simulink model "gm_DVBS"  (R2023b)
settings: Solver=FixedStepAuto  StartTime=0.0  StopTime=160000/fs  FixedStep=5e-9  RelTol=1e-3  EnableMultiTasking=on
undefined symbols (not defined in the file or in its folder): ctrlIn, fc, fs, iniStates, k, n, oneData, rb, Rcos, simDataIn, sourceData
libraries: simulink x29, hdlsllib x23, commdigbbndpm3 x4, commhdlblkcod x4, dspsrcs4 x3, whdledac x1, commsink2 x1, commcnvintrlv2 x1, commchan3 x1, dsphdlsigops2 x1, commcnvcod2 x1
(part 2 of 2)

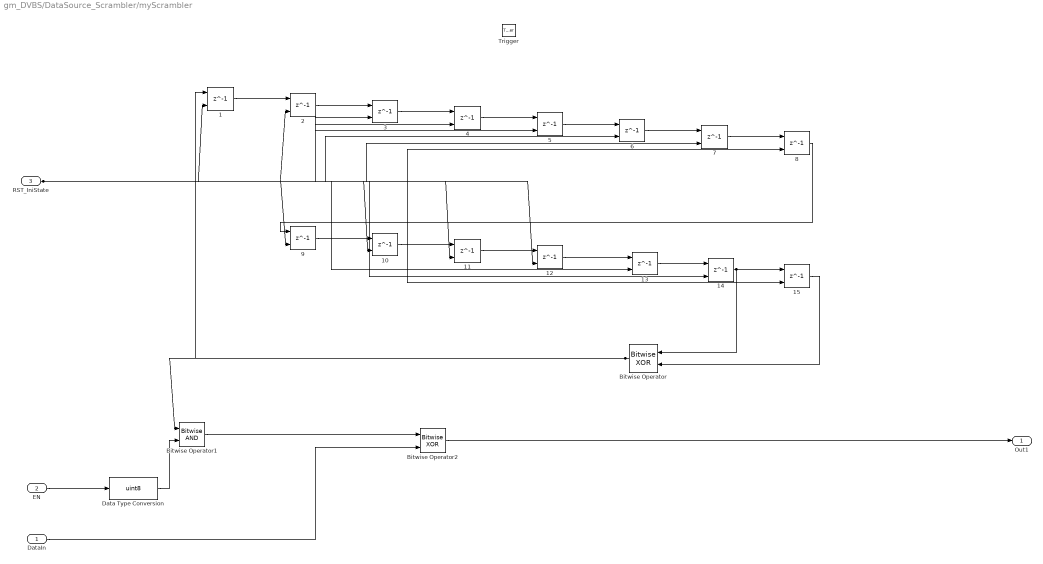
== system gm_DVBS/DataSource_Scrambler/myScrambler ==
  DataIn : Inport  OutDataTypeStr=uint8  PortDimensions=1
  EN : Inport  Port=2  OutDataTypeStr=boolean  PortDimensions=1
  RST_IniState : Inport  Port=3  OutDataTypeStr=boolean  PortDimensions=1
  Trigger : TriggerPort  VariantControl=(inherit)  PortDimensions=1  OutDataTypeStr=boolean
  1 : Delay  DelayLength=1  InitialCondition=iniStates(1)  ExternalReset=Level
      settings: InputPortMap=u0,r5
  10 : Delay  DelayLength=1  InitialCondition=iniStates(10)  ExternalReset=Level
      settings: InputPortMap=u0,r5
  11 : Delay  DelayLength=1  InitialCondition=iniStates(11)  ExternalReset=Level
      settings: InputPortMap=u0,r5
  12 : Delay  DelayLength=1  InitialCondition=iniStates(12)  ExternalReset=Level
      settings: InputPortMap=u0,r5
  13 : Delay  DelayLength=1  InitialCondition=iniStates(13)  ExternalReset=Level
      settings: InputPortMap=u0,r5
  14 : Delay  DelayLength=1  InitialCondition=iniStates(14)  ExternalReset=Level
      settings: InputPortMap=u0,r5
  15 : Delay  DelayLength=1  InitialCondition=iniStates(15)  ExternalReset=Level
      settings: InputPortMap=u0,r5
  2 : Delay  DelayLength=1  InitialCondition=iniStates(2)  ExternalReset=Level
      settings: InputPortMap=u0,r5
  3 : Delay  DelayLength=1  InitialCondition=iniStates(3)  ExternalReset=Level
      settings: InputPortMap=u0,r5
  4 : Delay  DelayLength=1  InitialCondition=iniStates(4)  ExternalReset=Level
      settings: InputPortMap=u0,r5
  5 : Delay  DelayLength=1  InitialCondition=iniStates(5)  ExternalReset=Level
      settings: InputPortMap=u0,r5
  6 : Delay  DelayLength=1  InitialCondition=iniStates(6)  ExternalReset=Level
      settings: InputPortMap=u0,r5
  7 : Delay  DelayLength=1  InitialCondition=iniStates(7)  ExternalReset=Level
      settings: InputPortMap=u0,r5
  8 : Delay  DelayLength=1  InitialCondition=iniStates(8)  ExternalReset=Level
      settings: InputPortMap=u0,r5
  9 : Delay  DelayLength=1  InitialCondition=iniStates(9)  ExternalReset=Level
      settings: InputPortMap=u0,r5
  Bitwise Operator : simulink/Logic and Bit Operations/Bitwise Operator  logicop=XOR  UseBitMask=off  NumInputPorts=2  BitMask=bin2dec('11011001')  BitMaskRealWorld=Stored Integer
  Bitwise Operator1 : simulink/Logic and Bit Operations/Bitwise Operator  logicop=AND  UseBitMask=off  NumInputPorts=2  BitMask=bin2dec('11011001')  BitMaskRealWorld=Stored Integer
  Bitwise Operator2 : simulink/Logic and Bit Operations/Bitwise Operator  logicop=XOR  UseBitMask=off  NumInputPorts=2  BitMask=bin2dec('11011001')  BitMaskRealWorld=Stored Integer
  Data Type Conversion : DataTypeConversion  OutDataTypeStr=uint8  SaturateOnIntegerOverflow=off  RndMeth=Floor
  Out1 : Outport  InitialOutput=0
  wires:
  DataIn/1 -> Bitwise Operator2/2
  EN/1 -> Data Type Conversion/1
  RST_IniState/1 -> 14/2, 13/2, 12/2, 11/2, 10/2, 9/2, 8/2, 7/2, 6/2, 5/2, 4/2, 3/2, 2/2, 1/2, 15/2
  Bitwise Operator/1 -> Bitwise Operator1/1, 1/1
  Bitwise Operator1/1 -> Bitwise Operator2/1
  Bitwise Operator2/1 -> Out1/1
  Data Type Conversion/1 -> Bitwise Operator1/2
  15/1 -> Bitwise Operator/2
  1/1 -> 2/1
  2/1 -> 3/1
  3/1 -> 4/1
  4/1 -> 5/1
  5/1 -> 6/1
  6/1 -> 7/1
  7/1 -> 8/1
  8/1 -> 9/1
  9/1 -> 10/1
  10/1 -> 11/1
  11/1 -> 12/1
  12/1 -> 13/1
  13/1 -> 14/1
  14/1 -> Bitwise Operator/1, 15/1

== system gm_DVBS/DataSource_Scrambler/sigSource ==
  DataGenEn : Inport  OutDataTypeStr=boolean  PortDimensions=1  SampleTime=5e-09
  Enable : Inport  Port=2  OutDataTypeStr=boolean  SampleTime=5e-09
  1-D Lookup Table : Lookup_n-D  NumberOfTableDimensions=1  LookupTableObject=''  BreakpointsForDimension1=[0:18800-1]'  BreakpointsForDimension1FirstPoint=10  BreakpointsForDimension2FirstPoint=10  BreakpointsForDimension1Spacing=12  BreakpointsForDimension2Spacing=12  IndexSearchMethod=Evenly spaced points  Table=sourceData  InterpMethod=Flat  DiagnosticForOutOfRangeInput=Error  InternalRulePriority=Speed  OutDataTypeStr=uint8  RndMeth=Simplest
  DATA_IN : DataTypeConversion  OutDataTypeStr=fixdt(0,8,0)
  HDL Counter : Subsystem
      settings: MinAlgLoopOccurrences=on
  RS_Gen : Subsystem
  out_0_pipe : Delay  DelayLength=double(1)  InitialCondition=0
  out_1_pipe : Delay  DelayLength=double(1)  InitialCondition=0
  out_2_pipe : Delay  DelayLength=double(1)  InitialCondition=0
  out_3_pipe : Delay  DelayLength=double(1)  InitialCondition=0
  simStart : Outport  SampleTime=5e-09  InitialOutput=0
  simEnd : Outport  Port=2  SampleTime=5e-09  InitialOutput=0
  simEN : Outport  Port=3  SampleTime=5e-09  InitialOutput=0
  simDataIn : Outport  Port=4  SampleTime=5e-09  InitialOutput=0
  wires:
  Enable/1 -> HDL Counter/Enable, RS_Gen/1(Enable_out2)
  DataGenEn/1 -> HDL Counter/1(in0)
  1-D Lookup Table/1 -> DATA_IN/1
  DATA_IN/1 -> out_3_pipe/1
  HDL Counter/1(out0) -> 1-D Lookup Table/1
  RS_Gen/1(simStart) -> out_0_pipe/1
  RS_Gen/2(simEnd) -> out_1_pipe/1
  RS_Gen/3(simEN) -> out_2_pipe/1
  out_0_pipe/1 -> simStart/1
  out_1_pipe/1 -> simEnd/1
  out_2_pipe/1 -> simEN/1
  out_3_pipe/1 -> simDataIn/1

== system gm_DVBS/DataSource_Scrambler1/CLKdivide ==
  Constant : Constant  Value=8  VectorParams1D=off  OutDataTypeStr=uint8  SampleTime=1/fs
  Constant1 : Constant  Value=25  VectorParams1D=off  OutDataTypeStr=uint8  SampleTime=1/fs
  Delay : Delay  DelayLength=1
  Detect Rise Positive : hdlsllib/Logic and Bit Operations/Detect Rise Positive  vinit=0  OutDataTypeStr=boolean
  HDL Counter : hdlsllib/Sources/HDL Counter  CountType=Count limited  CountInit=1  CountStep=1  CountMax=8  CountFromType=Initial value  CountFrom=1  CountResetPort=off  CountLoadPort=off  CountEnbPort=on  CountDirPort=off  CountHitOutputPort=off  CountDataType=Unsigned  CountWordLen=8  CountFracLen=0  CountSampTime=1
  HDL Counter2 : hdlsllib/Sources/HDL Counter  CountType=Count limited  CountInit=1  CountStep=1  CountMax=25  CountFromType=Initial value  CountFrom=1  CountResetPort=off  CountLoadPort=off  CountEnbPort=off  CountDirPort=off  CountHitOutputPort=off  CountDataType=Unsigned  CountWordLen=8  CountFracLen=0  CountSampTime=1/fs
  Relational Operator : RelationalOperator  Operator===  OutDataTypeStr=boolean  InputSameDT=off
  Relational Operator1 : RelationalOperator  Operator===  OutDataTypeStr=boolean  InputSameDT=off
  DataGenEn : Outport  VectorParamsAs1DForOutWhenUnconnected=off
  BinEn : Outport  Port=2  VectorParamsAs1DForOutWhenUnconnected=off
  wires:
  Constant/1 -> Relational Operator1/2
  Detect Rise Positive/1 -> DataGenEn/1
  Relational Operator1/1 -> Detect Rise Positive/1
  HDL Counter/1 -> Relational Operator1/1
  HDL Counter2/1 -> Relational Operator/1
  Delay/1 -> BinEn/1
  Relational Operator/1 -> HDL Counter/1, Delay/1
  Constant1/1 -> Relational Operator/2

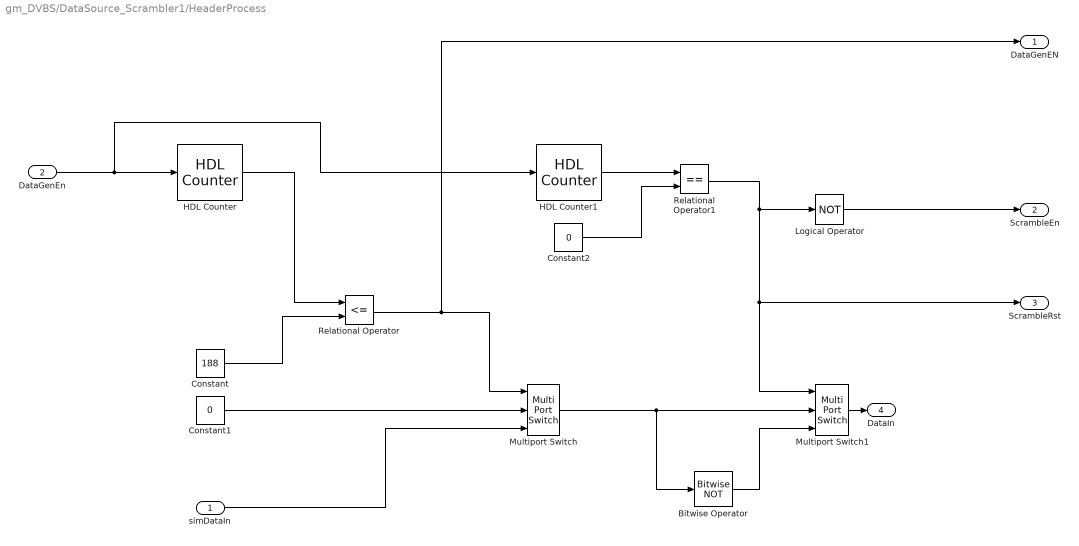
== system gm_DVBS/DataSource_Scrambler1/HeaderProcess ==
  simDataIn : Inport
  DataGenEn : Inport  Port=2
  Bitwise Operator : simulink/Logic and Bit Operations/Bitwise Operator  logicop=NOT  UseBitMask=off  BitMask=bin2dec('11011001')  BitMaskRealWorld=Stored Integer
  Constant : Constant  Value=188  OutDataTypeStr=uint8  SampleTime=1/fs
  Constant1 : Constant  Value=0  OutDataTypeStr=uint8
  Constant2 : Constant  Value=0  OutDataTypeStr=uint8
  HDL Counter : hdlsllib/Sources/HDL Counter  CountType=Count limited  CountInit=1  CountStep=1  CountMax=n  CountFromType=Initial value  CountFrom=1  CountResetPort=off  CountLoadPort=off  CountEnbPort=on  CountDirPort=off  CountHitOutputPort=off  CountDataType=Unsigned  CountWordLen=8  CountFracLen=0  CountSampTime=1/fs
  HDL Counter1 : hdlsllib/Sources/HDL Counter  CountType=Count limited  CountInit=0  CountStep=1  CountMax=n*8-1  CountFromType=Initial value  CountFrom=0  CountResetPort=off  CountLoadPort=off  CountEnbPort=on  CountDirPort=off  CountHitOutputPort=off  CountDataType=Unsigned  CountWordLen=16  CountFracLen=0  CountSampTime=1/fs
  Logical Operator : Logic  Operator=NOT  AllPortsSameDT=off  OutDataTypeStr=boolean
  Multiport Switch : MultiPortSwitch  DataPortOrder=Specify indices  DataPortIndices={0,1}  OutDataTypeStr=uint8  SaturateOnIntegerOverflow=off  InputSameDT=off
  Multiport Switch1 : MultiPortSwitch  DataPortOrder=Specify indices  DataPortIndices={0,1}  OutDataTypeStr=uint8  SaturateOnIntegerOverflow=off  InputSameDT=off
  Relational Operator : RelationalOperator  Operator=<=  OutDataTypeStr=boolean  InputSameDT=off
  Relational Operator1 : RelationalOperator  Operator===  OutDataTypeStr=boolean  InputSameDT=off
  DataGenEN : Outport  VectorParamsAs1DForOutWhenUnconnected=off
  ScrambleEn : Outport  Port=2  VectorParamsAs1DForOutWhenUnconnected=off
  ScrambleRst : Outport  Port=3  VectorParamsAs1DForOutWhenUnconnected=off
  DataIn : Outport  Port=4
  wires:
  DataGenEn/1 -> HDL Counter/1, HDL Counter1/1
  simDataIn/1 -> Multiport Switch/3
  Logical Operator/1 -> ScrambleEn/1
  Constant1/1 -> Multiport Switch/2
  Constant2/1 -> Relational Operator1/2
  Constant/1 -> Relational Operator/2
  Relational Operator1/1 -> Logical Operator/1, Multiport Switch1/1, ScrambleRst/1
  Relational Operator/1 -> Multiport Switch/1, DataGenEN/1
  HDL Counter1/1 -> Relational Operator1/1
  HDL Counter/1 -> Relational Operator/1
  Multiport Switch/1 -> Multiport Switch1/2, Bitwise Operator/1
  Bitwise Operator/1 -> Multiport Switch1/3
  Multiport Switch1/1 -> DataIn/1

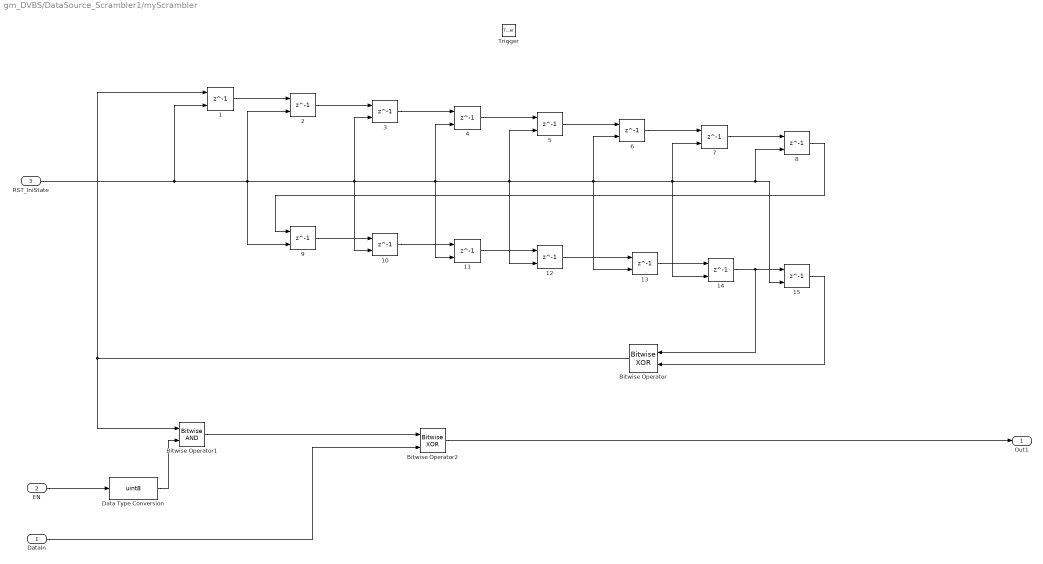
== system gm_DVBS/DataSource_Scrambler1/myScrambler ==
  DataIn : Inport  OutDataTypeStr=uint8
  EN : Inport  Port=2  OutDataTypeStr=boolean
  RST_IniState : Inport  Port=3  OutDataTypeStr=boolean
  Trigger : TriggerPort  VariantControl=Variant  PortDimensions=1
  1 : Delay  DelayLength=1  InitialCondition=iniStates(1)  ExternalReset=Level
      settings: InputPortMap=u0,r5
  10 : Delay  DelayLength=1  InitialCondition=iniStates(10)  ExternalReset=Level
      settings: InputPortMap=u0,r5
  11 : Delay  DelayLength=1  InitialCondition=iniStates(11)  ExternalReset=Level
      settings: InputPortMap=u0,r5
  12 : Delay  DelayLength=1  InitialCondition=iniStates(12)  ExternalReset=Level
      settings: InputPortMap=u0,r5
  13 : Delay  DelayLength=1  InitialCondition=iniStates(13)  ExternalReset=Level
      settings: InputPortMap=u0,r5
  14 : Delay  DelayLength=1  InitialCondition=iniStates(14)  ExternalReset=Level
      settings: InputPortMap=u0,r5
  15 : Delay  DelayLength=1  InitialCondition=iniStates(15)  ExternalReset=Level
      settings: InputPortMap=u0,r5
  2 : Delay  DelayLength=1  InitialCondition=iniStates(2)  ExternalReset=Level
      settings: InputPortMap=u0,r5
  3 : Delay  DelayLength=1  InitialCondition=iniStates(3)  ExternalReset=Level
      settings: InputPortMap=u0,r5
  4 : Delay  DelayLength=1  InitialCondition=iniStates(4)  ExternalReset=Level
      settings: InputPortMap=u0,r5
  5 : Delay  DelayLength=1  InitialCondition=iniStates(5)  ExternalReset=Level
      settings: InputPortMap=u0,r5
  6 : Delay  DelayLength=1  InitialCondition=iniStates(6)  ExternalReset=Level
      settings: InputPortMap=u0,r5
  7 : Delay  DelayLength=1  InitialCondition=iniStates(7)  ExternalReset=Level
      settings: InputPortMap=u0,r5
  8 : Delay  DelayLength=1  InitialCondition=iniStates(8)  ExternalReset=Level
      settings: InputPortMap=u0,r5
  9 : Delay  DelayLength=1  InitialCondition=iniStates(9)  ExternalReset=Level
      settings: InputPortMap=u0,r5
  Bitwise Operator : simulink/Logic and Bit Operations/Bitwise Operator  logicop=XOR  UseBitMask=off  NumInputPorts=2  BitMask=bin2dec('11011001')  BitMaskRealWorld=Stored Integer
  Bitwise Operator1 : simulink/Logic and Bit Operations/Bitwise Operator  logicop=AND  UseBitMask=off  NumInputPorts=2  BitMask=bin2dec('11011001')  BitMaskRealWorld=Stored Integer
  Bitwise Operator2 : simulink/Logic and Bit Operations/Bitwise Operator  logicop=XOR  UseBitMask=off  NumInputPorts=2  BitMask=bin2dec('11011001')  BitMaskRealWorld=Stored Integer
  Data Type Conversion : DataTypeConversion  OutDataTypeStr=uint8  SaturateOnIntegerOverflow=off  RndMeth=Floor
  Out1 : Outport  InitialOutput=0
  wires:
  Data Type Conversion/1 -> Bitwise Operator1/2
  RST_IniState/1 -> 3/2, 5/2, 6/2, 7/2, 15/2, 8/2, 14/2, 13/2, 12/2, 11/2, 4/2, 10/2, 9/2, 2/2, 1/2
  8/1 -> 9/1
  Bitwise Operator2/1 -> Out1/1
  DataIn/1 -> Bitwise Operator2/2
  Bitwise Operator1/1 -> Bitwise Operator2/1
  EN/1 -> Data Type Conversion/1
  Bitwise Operator/1 -> 1/1, Bitwise Operator1/1
  15/1 -> Bitwise Operator/2
  14/1 -> 15/1, Bitwise Operator/1
  13/1 -> 14/1
  12/1 -> 13/1
  11/1 -> 12/1
  10/1 -> 11/1
  9/1 -> 10/1
  7/1 -> 8/1
  6/1 -> 7/1
  5/1 -> 6/1
  4/1 -> 5/1
  3/1 -> 4/1
  2/1 -> 3/1
  1/1 -> 2/1

== system gm_DVBS/DataSource_Scrambler1/sigSource ==
  DataGenEn : Inport
  Enable : EnablePort
  1-D Lookup Table : Lookup_n-D  NumberOfTableDimensions=1  LookupTableObject=''  BreakpointsForDimension1=[0:18800-1]'  BreakpointsForDimension1FirstPoint=10  BreakpointsForDimension2FirstPoint=10  BreakpointsForDimension1Spacing=12  BreakpointsForDimension2Spacing=12  IndexSearchMethod=Evenly spaced points  Table=sourceData  InterpMethod=Flat  DiagnosticForOutOfRangeInput=Error  InternalRulePriority=Speed  OutDataTypeStr=uint8  RndMeth=Simplest
  DATA_IN : DataTypeConversion  OutDataTypeStr=inDataType  SaturateOnIntegerOverflow=off  RndMeth=Floor
  Detect Rise Positive : hdlsllib/Logic and Bit Operations/Detect Rise Positive  vinit=0  OutDataTypeStr=boolean
  Detect Rise Positive1 : hdlsllib/Logic and Bit Operations/Detect Rise Positive  vinit=0  OutDataTypeStr=boolean
  HDL Counter : hdlsllib/Sources/HDL Counter  CountType=Count limited  CountInit=0  CountStep=1  CountMax=18800-1  CountFromType=Initial value  CountFrom=0  CountResetPort=off  CountLoadPort=off  CountEnbPort=on  CountDirPort=off  CountHitOutputPort=off  CountDataType=Unsigned  CountWordLen=32  CountFracLen=0  CountSampTime=1/fs
  RS_Gen : Subsystem
  Subsystem : Subsystem  Commented=on
  simStart : Outport  InitialOutput=0
  simEnd : Outport  Port=2  InitialOutput=0
  simEN : Outport  Port=3  InitialOutput=0
  simDataIn : Outport  Port=4  InitialOutput=0
  wires:
  Detect Rise Positive1/1 -> simEnd/1
  Detect Rise Positive/1 -> simStart/1
  DATA_IN/1 -> simDataIn/1
  RS_Gen/3(simEN) -> simEN/1
  RS_Gen/2(simEnd) -> Detect Rise Positive1/1
  RS_Gen/1(simStart) -> Detect Rise Positive/1
  DataGenEn/1 -> RS_Gen/Trigger, HDL Counter/1
  HDL Counter/1 -> 1-D Lookup Table/1
  1-D Lookup Table/1 -> DATA_IN/1

== system gm_DVBS/Interleaver/Con_Interleaver ==
  In1 : Inport
  Trigger : TriggerPort  VariantControl=Variant  PortDimensions=1
  Convolutional Interleaver : commcnvintrlv2/Convolutional Interleaver  N=12  B=17  ic=0
      settings: LibrarySourceBlock=|
      | commhdlinterleave/Convolutional
      | Interleaver
  Out1 : Outport  InitialOutput=0
  wires:
  Convolutional Interleaver/1 -> Out1/1
  In1/1 -> Convolutional Interleaver/1

== system gm_DVBS/QPSK/QPSK_Modulation ==
  In1 : Inport
  Add : Sum  Inputs=+-
  Complex to Real-Imag : ComplexToRealImag
  Cosine : Sin  Frequency=fc*2*pi  Phase=pi/2  SampleTime=1/fs
  Discrete FIR Filter : DiscreteFir  Coefficients=Rcos
  Discrete FIR Filter1 : DiscreteFir  Coefficients=Rcos
  Product : Product
  Product1 : Product
  QPSK Modulator Baseband : commdigbbndpm3/QPSK Modulator Baseband  InType=Bit  Enc=Gray  Ph=pi/4  outDtype=double  outWordLen=16  outUDDataType=sfix(16)  outFracLenMode=Best precision  outFracLen=15  outDataTypeStr=double  outLastDataTypeStr=double
      settings: LibrarySourceBlock=|
      | commhdldigbbndpm/QPSK
      | Modulator
      | Baseband
  Sign : Signum  Commented=through
  Sign1 : Signum  Commented=through
  Sine : Sin  Frequency=fc*2*pi  SampleTime=1/fs
  Out1 : Outport
  Out2 : Outport  Port=2  VectorParamsAs1DForOutWhenUnconnected=off
  wires:
  In1/1 -> QPSK Modulator Baseband/1
  Sign1/1 -> Discrete FIR Filter1/1
  Complex to Real-Imag/1 -> Sign/1
  Discrete FIR Filter/1 -> Product/1
  Add/1 -> Out1/1
  QPSK Modulator Baseband/1 -> Complex to Real-Imag/1, Out2/1
  Product/1 -> Add/1
  Product1/1 -> Add/2
  Discrete FIR Filter1/1 -> Product1/2
  Sign/1 -> Discrete FIR Filter/1
  Sine/1 -> Product1/1
  Cosine/1 -> Product/2
  Complex to Real-Imag/2 -> Sign1/1

== system gm_DVBS/QPSK/Subsystem ==
  In1 : Inport
  Cos : Sin  Frequency=fc*2*pi  Phase=pi/2  SampleTime=1/fs
  Discrete FIR Filter : DiscreteFir  Coefficients=Rcos
  Discrete FIR Filter1 : DiscreteFir  Coefficients=Rcos
  Product : Product
  Product1 : Product
  QPSK Demodulator Baseband : commdigbbndpm3/QPSK Demodulator Baseband  OutType=Integer  DecType=Hard decision  VarSource=Dialog  Variance=1  Dec=Gray  Ph=pi/4  outDtype1=Inherit via internal rule  outDtype2=Inherit via internal rule  derotateFactorWordLen=16  derotateFactorDataTypeStr=Inherit: Same word length as input  derotateFactorLastDataTypeStr=Inherit: Same word length as input
      settings: LibrarySourceBlock=|
      | commhdldigbbndpm/QPSK
      | Demodulator
      | Baseband
  Real-Imag to Complex : RealImagToComplex
  Sin : Sin  Frequency=fc*2*pi  SampleTime=1/fs
  Out1 : Outport
  wires:
  Discrete FIR Filter/1 -> Real-Imag to Complex/2
  Discrete FIR Filter1/1 -> Real-Imag to Complex/1
  QPSK Demodulator Baseband/1 -> Out1/1
  Real-Imag to Complex/1 -> QPSK Demodulator Baseband/1
  Product1/1 -> Discrete FIR Filter/1
  Product/1 -> Discrete FIR Filter1/1
  Sin/1 -> Product1/1
  Cos/1 -> Product/2
  In1/1 -> Product/1, Product1/2

== system gm_DVBS/RS_Enc/RS ==
  RS_In : Inport  OutDataTypeStr=uint8
  RS_Start : Inport  Port=2  OutDataTypeStr=boolean
  RS_End : Inport  Port=3  OutDataTypeStr=boolean
  RS_VLD : Inport  Port=4  OutDataTypeStr=boolean
  Trigger : TriggerPort  VariantControl=Variant  PortDimensions=1
  Integer-Input RS Encoder HDL Optimized : commhdlblkcod/Integer-Input RS Encoder HDL Optimized  CodewordLength=n  MessageLength=k  PrimitivePolynomialSource=Property  PrimitivePolynomial=[1 0 0 0 1 1 1 0 1]  PuncturePatternSource=None  PuncturePattern=[ ones( 2, 1 ); zeros( 2, 1 ) ]  BSource=Property  B=0  SimulateUsing=Code generation
  Terminator : Terminator
  Terminator1 : Terminator
  Terminator2 : Terminator
  RS_Out : Outport  OutDataTypeStr=uint8  InitialOutput=0
  wires:
  Integer-Input RS Encoder HDL Optimized/4 -> Terminator2/1
  Integer-Input RS Encoder HDL Optimized/3 -> Terminator1/1
  Integer-Input RS Encoder HDL Optimized/2 -> Terminator/1
  RS_VLD/1 -> Integer-Input RS Encoder HDL Optimized/4
  RS_End/1 -> Integer-Input RS Encoder HDL Optimized/3
  RS_Start/1 -> Integer-Input RS Encoder HDL Optimized/2
  Integer-Input RS Encoder HDL Optimized/1 -> RS_Out/1
  RS_In/1 -> Integer-Input RS Encoder HDL Optimized/1

== system gm_DVBS/Subsystem/Subsystem ==
  Constant : Constant  OutDataTypeStr=boolean  SampleTime=1/fs
  NCO : dsphdlsigops2/NCO  PhaseIncrementSource=Property  PhaseIncrement=phInc  PhaseOffsetSource=Property  PhaseOffset=0  DitherSource=Property  NumDitherBits=4  SamplesPerFrame=1  LUTCompress=on  ResetAction=off  Waveform=Sine and cosine  PhasePort=off  SimulateUsing=Code generation  AccumulatorWL=N  PhaseQuantization=on  NumQuantizerAccumulatorBits=Q  OutputDataType=Binary point scaling  OutputWL=32  OutputFL=30
      settings: LibrarySourceBlock=dsphdlsrcs2/NCO
  sin : Outport
  cos : Outport  Port=2
  vld : Outport  Port=3
  wires:
  NCO/2 -> cos/1
  NCO/3 -> vld/1
  NCO/1 -> sin/1
  Constant/1 -> NCO/1

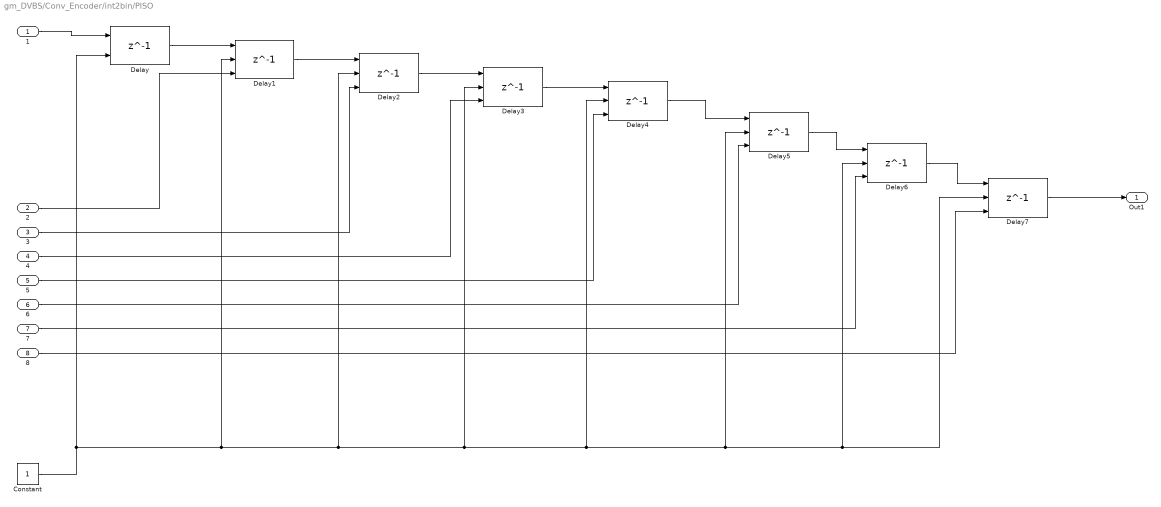
== system gm_DVBS/Conv_Encoder/int2bin/PISO ==
  1 : Inport
  2 : Inport  Port=2
  3 : Inport  Port=3
  4 : Inport  Port=4
  5 : Inport  Port=5
  6 : Inport  Port=6
  7 : Inport  Port=7
  8 : Inport  Port=8
  Constant : Constant  OutDataTypeStr=boolean  SampleTime=1
  Delay : Delay  DelayLength=1  InitialCondition=0  ShowEnablePort=on  UseCircularBuffer=on  SampleTime=1
      settings: InputPortMap=u0,e6
  Delay{1..7} (7 alike) : Delay  DelayLength=1  InitialConditionSource=Input port  InitialCondition=0  ShowEnablePort=on  UseCircularBuffer=on  SampleTime=1
      settings: InputPortMap=u0,e6,p4
  Out1 : Outport
  wires:
  5/1 -> Delay4/3
  Delay7/1 -> Out1/1
  Delay6/1 -> Delay7/1
  6/1 -> Delay5/3
  8/1 -> Delay7/3
  7/1 -> Delay6/3
  Delay4/1 -> Delay5/1
  Delay5/1 -> Delay6/1
  Constant/1 -> Delay3/2, Delay7/2, Delay6/2, Delay5/2, Delay4/2, Delay2/2, Delay1/2, Delay/2
  Delay3/1 -> Delay4/1
  4/1 -> Delay3/3
  3/1 -> Delay2/3
  2/1 -> Delay1/3
  Delay2/1 -> Delay3/1
  Delay1/1 -> Delay2/1
  Delay/1 -> Delay1/1
  1/1 -> Delay/1

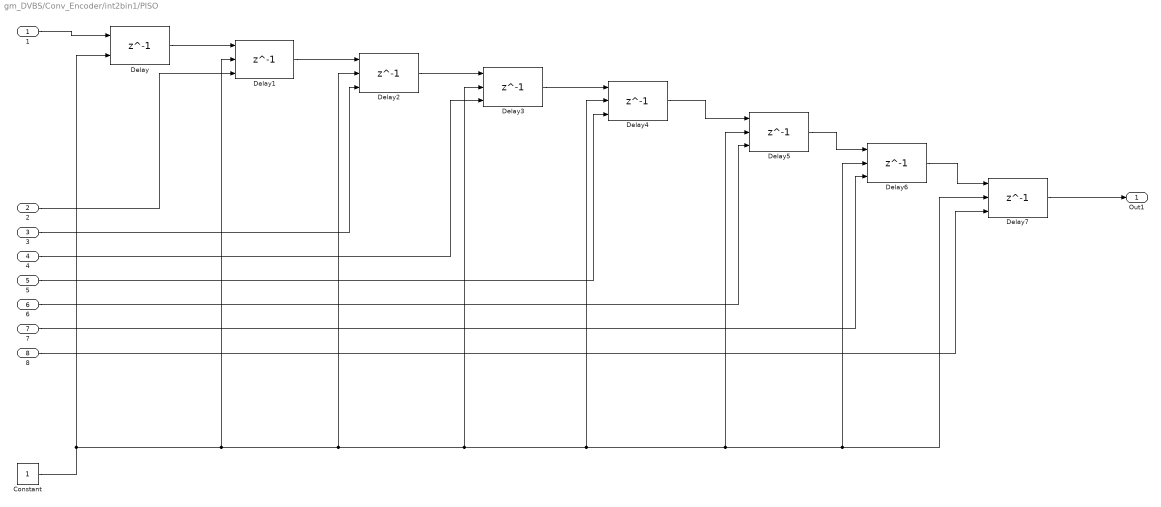
== system gm_DVBS/Conv_Encoder/int2bin1/PISO ==
  1 : Inport
  2 : Inport  Port=2
  3 : Inport  Port=3
  4 : Inport  Port=4
  5 : Inport  Port=5
  6 : Inport  Port=6
  7 : Inport  Port=7
  8 : Inport  Port=8
  Constant : Constant  OutDataTypeStr=boolean  SampleTime=1
  Delay : Delay  DelayLength=1  InitialCondition=0  ShowEnablePort=on  UseCircularBuffer=on  SampleTime=1
      settings: InputPortMap=u0,e6
  Delay{1..7} (7 alike) : Delay  DelayLength=1  InitialConditionSource=Input port  InitialCondition=0  ShowEnablePort=on  UseCircularBuffer=on  SampleTime=1
      settings: InputPortMap=u0,e6,p4
  Out1 : Outport
  wires:
  5/1 -> Delay4/3
  Delay7/1 -> Out1/1
  Delay6/1 -> Delay7/1
  6/1 -> Delay5/3
  8/1 -> Delay7/3
  7/1 -> Delay6/3
  Delay4/1 -> Delay5/1
  Delay5/1 -> Delay6/1
  Constant/1 -> Delay3/2, Delay7/2, Delay6/2, Delay5/2, Delay4/2, Delay2/2, Delay1/2, Delay/2
  Delay3/1 -> Delay4/1
  4/1 -> Delay3/3
  3/1 -> Delay2/3
  2/1 -> Delay1/3
  Delay2/1 -> Delay3/1
  Delay1/1 -> Delay2/1
  Delay/1 -> Delay1/1
  1/1 -> Delay/1

== system gm_DVBS/DataSource_Scrambler/CLKdivide/Detect Rise Positive ==
  note: Edge
  note: U(k)
  U : Inport  OutDataTypeStr=boolean  SampleTime=5e-09
  Delay Input1 : UnitDelay  Description=Store in Global RAM  DisableCoverage=on  InitialCondition=vinit  SampleTime=-1  HasFrameUpgradeWarning=on
  FixPt Relational Operator : RelationalOperator  Operator=>  OutDataTypeStr=boolean  ZeroCross=off  InputSameDT=off
  Positive : Subsystem  mask(Compare To Zero){relop=>, OutDataTypeStr=boolean, ZeroCross=off}
      mask prompts: relop "Simulink:masks:Operator_MP"; OutDataTypeStr "Simulink:masks:OutputDataType_MP"; ZeroCross "Simulink:masks:EnableZerocrossingDetection_MP"
      mask help: Simulink:masks:CompareToZero_MD
      mask init:
      | OutDataTypeStr = 'boolean';
      | ZeroCross = 'off';
      | blkName = 'DVBS/DataSource_Scrambler/CLKdivide/Detect Rise\nPositive/Positive';
      | relop = '>';
      | setValue = 'boolean';
      mask TypeOptions relop: == | ~= | < | <= | >= | >
      mask TypeOptions OutDataTypeStr: Simulink:masks:uint8 | Simulink:masks:boolean
      mask Callback ZeroCross: sl('zeroCrossEnable', gcbh);
      mask Display: disp([relop,' 0'])
  Y : Outport  SampleTime=5e-09
  wires:
  U/1 -> Positive/1(u)
  Delay Input1/1 -> FixPt Relational Operator/2
  FixPt Relational Operator/1 -> Y/1
  Positive/1(y) -> FixPt Relational Operator/1, Delay Input1/1

== system gm_DVBS/DataSource_Scrambler/Detect Rise Positive/Positive ==
  u : Inport  OutDataTypeStr=boolean  SampleTime=5e-09
  Compare : RelationalOperator  Operator=>  OutDataTypeStr=boolean  ZeroCross=off
  Constant : Constant  DisableCoverage=on  Value=0  OutDataTypeStr=Inherit: Inherit via back propagation  SampleTime=-1  PreserveConstantTs=on
  y : Outport  SampleTime=5e-09
  wires:
  u/1 -> Compare/1
  Compare/1 -> y/1
  Constant/1 -> Compare/2

== system gm_DVBS/DataSource_Scrambler/Detect Rise Positive1/Positive ==
  u : Inport  OutDataTypeStr=boolean  SampleTime=5e-09
  Compare : RelationalOperator  Operator=>  OutDataTypeStr=boolean  ZeroCross=off
  Constant : Constant  DisableCoverage=on  Value=0  OutDataTypeStr=Inherit: Inherit via back propagation  SampleTime=-1  PreserveConstantTs=on
  y : Outport  SampleTime=5e-09
  wires:
  u/1 -> Compare/1
  Compare/1 -> y/1
  Constant/1 -> Compare/2

== system gm_DVBS/DataSource_Scrambler/sigSource/HDL Counter ==
  in0 : Inport  OutDataTypeStr=boolean  SampleTime=5e-09
  Enable_out2 : EnablePort  OutDataTypeStr=boolean
  HDL Counter : hdlsllib/Sources/HDL Counter  CountType=Count limited  CountInit=0  CountStep=1  CountMax=18800-1  CountFromType=Initial value  CountFrom=0  CountResetPort=off  CountLoadPort=off  CountEnbPort=on  CountDirPort=off  CountHitOutputPort=off  CountDataType=Unsigned  CountWordLen=32  CountFracLen=0  CountSampTime=1/fs
  out0 : Outport  OutDataTypeStr=uint32  SampleTime=5e-09  InitialOutput=0
  wires:
  HDL Counter/1 -> out0/1
  in0/1 -> HDL Counter/1

== system gm_DVBS/DataSource_Scrambler/sigSource/RS_Gen ==
  Enable_out2 : Inport  OutDataTypeStr=boolean  SampleTime=5e-09
  Constant : Constant  Value=188  OutDataTypeStr=uint16  SampleTime=5e-09
  DATA_IN1 : DataTypeConversion  OutDataTypeStr=boolean  SampleTime=5e-09  SaturateOnIntegerOverflow=off  RndMeth=Floor
  DATA_IN2 : DataTypeConversion  OutDataTypeStr=boolean  SampleTime=5e-09  SaturateOnIntegerOverflow=off  RndMeth=Floor
  DATA_IN3 : DataTypeConversion  OutDataTypeStr=boolean  SampleTime=5e-09  SaturateOnIntegerOverflow=off  RndMeth=Floor
  MATLAB Function : Subsystem
      settings: MinAlgLoopOccurrences=on
  simStart : Outport  SampleTime=5e-09  InitialOutput=0
  simEnd : Outport  Port=2  SampleTime=5e-09  InitialOutput=0
  simEN : Outport  Port=3  SampleTime=5e-09  InitialOutput=0
  wires:
  Constant/1 -> MATLAB Function/1(in0)
  DATA_IN1/1 -> simEN/1
  DATA_IN2/1 -> simStart/1
  DATA_IN3/1 -> simEnd/1
  MATLAB Function/1(out0) -> DATA_IN1/1
  MATLAB Function/2(out1) -> DATA_IN2/1
  MATLAB Function/3(out2) -> DATA_IN3/1
  Enable_out2/1 -> MATLAB Function/Enable

== system gm_DVBS/DataSource_Scrambler1/sigSource/RS_Gen ==
  Trigger : TriggerPort  VariantControl=(inherit)  PortDimensions=1
  Constant : Constant  Value=204  OutDataTypeStr=uint16  SampleTime=-1
  DATA_IN1 : DataTypeConversion  OutDataTypeStr=boolean  SaturateOnIntegerOverflow=off  RndMeth=Floor
  DATA_IN2 : DataTypeConversion  OutDataTypeStr=boolean  SaturateOnIntegerOverflow=off  RndMeth=Floor
  DATA_IN3 : DataTypeConversion  OutDataTypeStr=boolean  SaturateOnIntegerOverflow=off  RndMeth=Floor
  MATLAB Function : MATLAB Function  TreatAsAtomicUnit=on
  simStart : Outport  InitialOutput=0
  simEnd : Outport  Port=2  InitialOutput=0
  simEN : Outport  Port=3  InitialOutput=0
  wires:
  MATLAB Function/1(enable) -> DATA_IN1/1
  Constant/1 -> MATLAB Function/1(totalLength)
  DATA_IN2/1 -> simStart/1
  DATA_IN1/1 -> simEN/1
  DATA_IN3/1 -> simEnd/1
  MATLAB Function/2(start) -> DATA_IN2/1
  MATLAB Function/3(endSignal) -> DATA_IN3/1

== system gm_DVBS/DataSource_Scrambler1/sigSource/Subsystem ==
  enb : Inport
  1-D Lookup Table1 : Lookup_n-D  NumberOfTableDimensions=1  LookupTableObject=''  BreakpointsForDimension1=[0:1020-1]'  BreakpointsForDimension1FirstPoint=10  BreakpointsForDimension2FirstPoint=10  BreakpointsForDimension1Spacing=12  BreakpointsForDimension2Spacing=12  IndexSearchMethod=Evenly spaced points  Table=oneData  InterpMethod=Flat  DiagnosticForOutOfRangeInput=Error  InternalRulePriority=Speed  OutDataTypeStr=uint8  RndMeth=Simplest
  DATA_IN4 : DataTypeConversion  OutDataTypeStr=inDataType  SaturateOnIntegerOverflow=off  RndMeth=Floor
  HDL Counter1 : hdlsllib/Sources/HDL Counter  CountType=Count limited  CountInit=0  CountStep=1  CountMax=1020  CountFromType=Initial value  CountFrom=0  CountResetPort=off  CountLoadPort=off  CountEnbPort=on  CountDirPort=off  CountHitOutputPort=off  CountDataType=Unsigned  CountWordLen=32  CountFracLen=0  CountSampTime=1/fs
  Out1 : Outport
  wires:
  HDL Counter1/1 -> 1-D Lookup Table1/1
  DATA_IN4/1 -> Out1/1
  enb/1 -> HDL Counter1/1
  1-D Lookup Table1/1 -> DATA_IN4/1

== system gm_DVBS/DataSource_Scrambler/CLKdivide/Detect Rise Positive/Positive ==
  u : Inport  OutDataTypeStr=boolean  SampleTime=5e-09
  Compare : RelationalOperator  Operator=>  OutDataTypeStr=boolean  ZeroCross=off
  Constant : Constant  DisableCoverage=on  Value=0  OutDataTypeStr=Inherit: Inherit via back propagation  SampleTime=-1  PreserveConstantTs=on
  y : Outport  SampleTime=5e-09
  wires:
  u/1 -> Compare/1
  Compare/1 -> y/1
  Constant/1 -> Compare/2

== system gm_DVBS/DataSource_Scrambler/sigSource/RS_Gen/MATLAB Function ==
  in0 : Inport  OutDataTypeStr=uint16  SampleTime=5e-09
  Enable_out2 : EnablePort  OutDataTypeStr=boolean
  MATLAB Function : Subsystem
  out0 : Outport  OutDataTypeStr=uint8  SampleTime=5e-09  InitialOutput=0
  out1 : Outport  Port=2  OutDataTypeStr=uint8  SampleTime=5e-09  InitialOutput=0
  out2 : Outport  Port=3  OutDataTypeStr=uint8  SampleTime=5e-09  InitialOutput=0
  wires:
  MATLAB Function/1(enable) -> out0/1
  MATLAB Function/2(start) -> out1/1
  MATLAB Function/3(endSignal) -> out2/1
  in0/1 -> MATLAB Function/1(totalLength)

== system gm_DVBS/DataSource_Scrambler/sigSource/RS_Gen/MATLAB Function/MATLAB Function ==
  totalLength : Inport  OutDataTypeStr=uint16  PortDimensions=1  SampleTime=5e-09
  MATLAB Function : MATLAB Function  TreatAsAtomicUnit=on
  enable : Outport  SampleTime=5e-09  InitialOutput=0  VectorParamsAs1DForOutWhenUnconnected=off
  start : Outport  Port=2  SampleTime=5e-09  InitialOutput=0
  endSignal : Outport  Port=3  SampleTime=5e-09  InitialOutput=0
  wires:
  MATLAB Function/1(enable) -> enable/1
  MATLAB Function/2(start) -> start/1
  MATLAB Function/3(endSignal) -> endSignal/1
  totalLength/1 -> MATLAB Function/1(totalLength)

== matlab function gm_DVBS/Conv_Encoder/int2bin/uint8tobin ==
  data: input input; bitValue output
function bitValue = bitwiseOutput(input)
    % 逐bit输出输入数据的二进制表示
    bitValue=zeros(1,8);
    for i = 1:8
        bitValue(i) = bitget(input, i);
        
    end

end

== matlab function gm_DVBS/sigSource/MATLAB Function ==
  data: totalLength input; enable output; start output; endSignal output
function [enable, start, endSignal] = rsSignals(totalLength)
    % rsSignals Generate enable, start, and end signals for RS(188,204)
    %
    % Input:
    %   totalLength - Total number of cycles the signals are active
    %
    % Output:
    %   enable - Enable signal (1 during transmission, 0 otherwise) as uint8
    %   start - Start signal (1 at the first cycle, 0 otherwise) as uint8
    %   endSignal - End signal (1 at the last cycle, 0 otherwise) as uint8

    % Persistent variable to keep track of the current cycle, as uint8
    persistent cycle;
    if isempty(cycle)
        cycle = uint8(0);  % Initialize the cycle count
    end

    % Increment cycle count
    cycle = cycle + 1;

    % Generate start signal
    if cycle == 1
        start = uint8(1);
    else
        start = uint8(0);
    end

    % Generate enable signal
    if cycle > 0 && cycle <= totalLength
        enable = uint8(1);
    else
        enable = uint8(0);
    end

    % Generate end signal
    if cycle == 188
        endSignal = uint8(1);
    else
        endSignal = uint8(0);
    end

    % Reset cycle count after reaching total length
    if cycle >= totalLength
        cycle = uint8(0);
    end
end

== matlab function gm_DVBS/DataSource_Scrambler/sigSource/RS_Gen/MATLAB Function/MATLAB Function/MATLAB Function ==
  data: totalLength input; enable output; start output; endSignal output
function [enable, start, endSignal] = rsSignals(totalLength)
    % rsSignals Generate enable, start, and end signals for RS(188,204)
    %
    % Input:
    %   totalLength - Total number of cycles the signals are active
    %
    % Output:
    %   enable - Enable signal (1 during transmission, 0 otherwise) as uint8
    %   start - Start signal (1 at the first cycle, 0 otherwise) as uint8
    %   endSignal - End signal (1 at the last cycle, 0 otherwise) as uint8

    % Persistent variable to keep track of the current cycle, as uint8
    persistent cycle;
    if isempty(cycle)
        cycle = uint8(0);  % Initialize the cycle count
    end

    % Increment cycle count
    cycle = cycle + 1;

    % Generate start signal
    if cycle == 1
        start = uint8(1);
    else
        start = uint8(0);
    end

    % Generate enable signal
    if cycle > 0 && cycle <= totalLength
        enable = uint8(1);
    else
        enable = uint8(0);
    end

    % Generate end signal
    if cycle == 188
        endSignal = uint8(1);
        cycle=uint8(0);
    else
        endSignal = uint8(0);
    end

    % Reset cycle count after reaching total length
    % if cycle >= totalLength
    %     cycle = uint8(0);
    % end
end

== matlab function gm_DVBS/sigSource11/MATLAB Function ==
  data: totalLength input; enable output; start output; endSignal output
function [enable, start, endSignal] = rsSignals(totalLength)
    % rsSignals Generate enable, start, and end signals for RS(188,204)
    %
    % Input:
    %   totalLength - Total number of cycles the signals are active
    %
    % Output:
    %   enable - Enable signal (1 during transmission, 0 otherwise) as uint8
    %   start - Start signal (1 at the first cycle, 0 otherwise) as uint8
    %   endSignal - End signal (1 at the last cycle, 0 otherwise) as uint8

    % Persistent variable to keep track of the current cycle, as uint8
    persistent cycle;
    if isempty(cycle)
        cycle = uint8(0);  % Initialize the cycle count
    end

    % Increment cycle count
    cycle = cycle + 1;

    % Generate start signal
    if cycle == 1
        start = uint8(1);
    else
        start = uint8(0);
    end

    % Generate enable signal
    if cycle > 0 && cycle <= totalLength
        enable = uint8(1);
    else
        enable = uint8(0);
    end

    % Generate end signal
    if cycle == 188
        endSignal = uint8(1);
    else
        endSignal = uint8(0);
    end

    % Reset cycle count after reaching total length
    if cycle >= totalLength
        cycle = uint8(0);
    end
end

== matlab function gm_DVBS/DataSource_Scrambler1/sigSource/RS_Gen/MATLAB Function ==
  data: totalLength input; enable output; start output; endSignal output
function [enable, start, endSignal] = rsSignals(totalLength)
    % rsSignals Generate enable, start, and end signals for RS(188,204)
    %
    % Input:
    %   totalLength - Total number of cycles the signals are active
    %
    % Output:
    %   enable - Enable signal (1 during transmission, 0 otherwise) as uint8
    %   start - Start signal (1 at the first cycle, 0 otherwise) as uint8
    %   endSignal - End signal (1 at the last cycle, 0 otherwise) as uint8

    % Persistent variable to keep track of the current cycle, as uint8
    persistent cycle;
    if isempty(cycle)
        cycle = uint8(0);  % Initialize the cycle count
    end

    % Increment cycle count
    cycle = cycle + 1;

    % Generate start signal
    if cycle == 1
        start = uint8(1);
    else
        start = uint8(0);
    end

    % Generate enable signal
    if cycle > 0 && cycle <= totalLength
        enable = uint8(1);
    else
        enable = uint8(0);
    end

    % Generate end signal
    if cycle == 188
        endSignal = uint8(1);
    else
        endSignal = uint8(0);
    end

    % Reset cycle count after reaching total length
    if cycle >= totalLength
        cycle = uint8(0);
    end
end

== matlab function gm_DVBS/Conv_Encoder/int2bin1/uint8tobin ==
  data: input input; bitValue output
function bitValue = bitwiseOutput(input)
    % 逐bit输出输入数据的二进制表示
    bitValue=zeros(1,8);
    for i = 1:8
        bitValue(i) = bitget(input, i);
        
    end

end
